simulink model "simple_control_system"  (R2016b)
settings: Solver=VariableStepAuto  StartTime=0.0  StopTime=10.0  RelTol=1e-3
values from neighbouring files (symbols this model uses):
  Ks = 100    [simulink_parameter.m]
  taua = 1e-3    (= 0.001)    [simulink_parameter.m]
  taup = 100e-3    (= 0.1)    [simulink_parameter.m]
  taus = 100e-6    (= 0.0001)    [simulink_parameter.m]
settings Model: Creator=lapmint  LastModifiedBy=lapmint

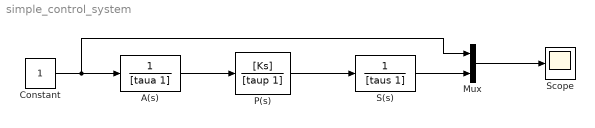
== system simple_control_system ==
  A(s) : TransferFcn  Denominator=[taua 1]
  Constant : Constant
  Mux : Mux  Inputs=2
  P(s) : TransferFcn  Numerator=[Ks]  Denominator=[taup 1]
  S(s) : TransferFcn  Denominator=[taus 1]
  Scope : Scope
  wires:
  A(s)/1 -> P(s)/1
  P(s)/1 -> S(s)/1
  Constant/1 -> Mux/1, A(s)/1
  S(s)/1 -> Mux/2
  Mux/1 -> Scope/1
